simulink model "eVTOL_HIL"  (R2024b)
settings: Solver=FixedStepAuto  StartTime=0.0  StopTime=inf  FixedStep=SAMPLE_TIME  RelTol=1e-3
values from neighbouring files (symbols this model uses):
  aDl =     [initdata.mat]
  aDr =     [initdata.mat]
  aDyn =     [initdata.mat]
  aLat =     [initdata.mat]
  aLon =     [initdata.mat]
  D = Prop.D    [EOM_dt_MC.m]    (also in EOM_get_alf_dt_de_prop_evtol.m = CD * QS)
  General = init_layoutdata    [EOM_dt_MC.m]    (also in build_optimized_CA.m; initdata.mat = ; initdata_HIL_eVTOL.m)
  mass = Con(3)    [EOM_get_alf_dt_de_prop_evtol.m]    (also in initdata.mat = 2255.54; initdata_HIL_eVTOL.m = 7)
  Motor = init_motor_evtol    [EOM_dt_MC.m]    (also in initdata.mat = []; initdata_HIL_eVTOL.m)
  Prop = init_propeller_evtol_new    [EOM_dt_MC.m]    (also in initdata_HIL_eVTOL.m)
  SAMPLE_TIME = 0.01    [initdata_HIL_eVTOL.m]
undefined symbols (not defined in the file or in its folder): aDa, aDe, asbhl20env, Environment, InitData, magnitude
libraries: simulink_extras x16, vrlib x8, matrix_library x6, sharedutil x6, aerolibwindfilters x4, sharedtransform x4, aerolibfltsims x3, instrumentseriallib x3, uavmavlinklib x3, aerolibasang x3, aerolibobsolete x2, aerolibanimutils x1
(part 4 of 4)

== system eVTOL_HIL/eVTOL Dynamic Model/airframe/force moment/aero F&M in body axis/nonunit value ==
  V : Inport
  pqr : Inport  Port=2
  alphaDot : Inport  Port=3
  CA : Constant  Value=General.MAC
  Demux2 : Demux  Outputs=3
      settings: DisplayOption=none
  Gain : Gain  Gain=2  SaturateOnIntegerOverflow=on  OutDataTypeStr=Inherit: Same as input  ParamDataTypeStr=Inherit: Same as input
  Mux18 : Mux  Inputs=3
  Product{1..4} (4 alike) : Product  Inputs=/**  SaturateOnIntegerOverflow=on  OutDataTypeStr=Inherit: Same as first input
  b : Constant  Value=General.b
  pqr_n : Outport  VectorParamsAs1DForOutWhenUnconnected=off
  alphaDot_n : Outport  Port=2  VectorParamsAs1DForOutWhenUnconnected=off
  wires:
  pqr/1 -> Demux2/1
  V/1 -> Gain/1
  Product4/1 -> Mux18/2
  Product2/1 -> Mux18/3
  Gain/1 -> Product1/1, Product2/1, Product3/1, Product4/1
  b/1 -> Product1/2, Product2/2
  Demux2/3 -> Product2/3  "r"
  Demux2/2 -> Product4/3  "q"
  Demux2/1 -> Product1/3  "p"
  CA/1 -> Product4/2, Product3/2
  Mux18/1 -> pqr_n/1
  Product1/1 -> Mux18/1
  alphaDot/1 -> Product3/3
  Product3/1 -> alphaDot_n/1

== system eVTOL_HIL/eVTOL Dynamic Model/Environment/Wind Models/Dryden Wind Turbulence Model (Continuous (+q -r))/RMS turbulence intensities/High Altitude Intensity ==
  h : Inport
  Medium/High Altitude Intensity : Interpolation_n-D  Table=sigma_vec'  ExtrapMethod=Clip  ValidIndexMayReachLast=on  OutDataTypeStr=double
  PreLook-Up Index Search (altitude) : PreLookup  BreakpointsData=h_vec  BeginIndexSearchUsingPreviousIndexResult=on  UseLastBreakpoint=on  FractionDataTypeStr=double
  PreLook-Up Index Search (prob of exceed) : PreLookup  BreakpointsData=[1:7]  BeginIndexSearchUsingPreviousIndexResult=on  UseLastBreakpoint=on  FractionDataTypeStr=double
  Probability of Exceedance : Constant  Value=TurbProb
  sigma_ug sigma_vg sigma_wg : Outport  InitialOutput=0  VectorParamsAs1DForOutWhenUnconnected=off
  wires:
  PreLook-Up Index Search (prob of exceed)/2 -> Medium/High Altitude Intensity/4
  PreLook-Up Index Search (prob of exceed)/1 -> Medium/High Altitude Intensity/3
  PreLook-Up Index Search (altitude)/2 -> Medium/High Altitude Intensity/2
  PreLook-Up Index Search (altitude)/1 -> Medium/High Altitude Intensity/1
  h/1 -> PreLook-Up Index Search (altitude)/1
  Medium/High Altitude Intensity/1 -> sigma_ug sigma_vg sigma_wg/1
  Probability of Exceedance/1 -> PreLook-Up Index Search (prob of exceed)/1

== system eVTOL_HIL/eVTOL Dynamic Model/Environment/Wind Models/Dryden Wind Turbulence Model (Continuous (+q -r))/RMS turbulence intensities/Low Altitude Intensity ==
  Windspeed at 20ft (6m) : Inport
  h : Inport  Port=2
  Limit Height h<1000ft : Saturate  UpperLimit=max_height_low  LowerLimit=0
  Low Altitude Intensity : Fcn  Expr=1/(0.177+0.000823*u(1))^0.4
  "sigma_ug, sigma_vg" : Product  InputSameDT=on  SaturateOnIntegerOverflow=on  OutDataTypeStr=Inherit: Same as first input
  "sigma_wg " : Gain  Gain=0.1  SaturateOnIntegerOverflow=on  OutDataTypeStr=Inherit: Same as input  ParamDataTypeStr=Inherit: Same as input
  sigma_ug sigma_vg : Outport  InitialOutput=0  VectorParamsAs1DForOutWhenUnconnected=off
  sigma_wg : Outport  Port=2  InitialOutput=0  VectorParamsAs1DForOutWhenUnconnected=off
  wires:
  "sigma_ug, sigma_vg"/1 -> sigma_ug sigma_vg/1
  h/1 -> Limit Height h<1000ft/1
  Low Altitude Intensity/1 -> "sigma_ug, sigma_vg"/1
  "sigma_wg "/1 -> sigma_wg/1, "sigma_ug, sigma_vg"/2
  Windspeed at 20ft (6m)/1 -> "sigma_wg "/1
  Limit Height h<1000ft/1 -> Low Altitude Intensity/1

== system eVTOL_HIL/eVTOL Dynamic Model/Environment/Wind Models/Dryden Wind Turbulence Model (Continuous (+q -r))/Select angular rates/Interpolate rates ==
  pgw_h&l : Inport
  qgw_h&l : Inport  Port=2
  rgw_h&l : Inport  Port=3
  DCM : Inport  Port=4
  Wind direction : Inport  Port=5
  Altitude : Inport  Port=6
  Action Port : ActionPort  PropagateVarSize=During execution  ActionPortLabel=else
  Mux : Mux  Inputs=3
  Mux1 : Mux  Inputs=3
  Product1 : Product  Inputs=**/  SaturateOnIntegerOverflow=on  OutDataTypeStr=Inherit: Same as first input
  Selector : Selector  InputPortWidth=2  IndexOptions=Index vector (dialog)  Indices=1  OutputSizes=1
  Selector1 : Selector  InputPortWidth=2  IndexOptions=Index vector (dialog)  Indices=1  OutputSizes=1
  Selector2 : Selector  InputPortWidth=2  IndexOptions=Index vector (dialog)  Indices=1  OutputSizes=1
  Selector3 : Selector  InputPortWidth=2  IndexOptions=Index vector (dialog)  Indices=2  OutputSizes=1
  Selector4 : Selector  InputPortWidth=2  IndexOptions=Index vector (dialog)  Indices=2  OutputSizes=1
  Selector5 : Selector  InputPortWidth=2  IndexOptions=Index vector (dialog)  Indices=2  OutputSizes=1
  Sum : Sum  Inputs=|-+  SaturateOnIntegerOverflow=on
  Sum1 : Sum  Inputs=|+-  SaturateOnIntegerOverflow=on
  Sum2 : Sum  Inputs=-+|  SaturateOnIntegerOverflow=on
  Sum3 : Sum  Inputs=++|  SaturateOnIntegerOverflow=on
  max_height_low : Constant  Value=max_height_low
  min_height_high : Constant  Value=min_height_high
  wind to body transformation : Subsystem
  pgw,qgw,rgw : Outport  InitialOutput=0  VectorParamsAs1DForOutWhenUnconnected=off
  wires:
  Mux/1 -> wind to body transformation/3(pg_l,qg_l,rg_l)
  DCM/1 -> wind to body transformation/1(DCM)
  wind to body transformation/1(pg,qg,rg) -> Sum3/1, Sum2/1
  Sum3/1 -> pgw,qgw,rgw/1
  Product1/1 -> Sum3/2
  Mux1/1 -> Sum2/2
  Sum2/1 -> Product1/1
  Sum1/1 -> Product1/2
  Sum/1 -> Product1/3
  Altitude/1 -> Sum1/1
  min_height_high/1 -> Sum/2
  max_height_low/1 -> Sum1/2, Sum/1
  Wind direction/1 -> wind to body transformation/2(Wind direction)
  Selector3/1 -> Mux1/1
  Selector4/1 -> Mux1/2
  Selector5/1 -> Mux1/3
  pgw_h&l/1 -> Selector/1, Selector3/1
  qgw_h&l/1 -> Selector4/1, Selector1/1
  rgw_h&l/1 -> Selector5/1, Selector2/1
  Selector/1 -> Mux/1
  Selector1/1 -> Mux/2
  Selector2/1 -> Mux/3

== system eVTOL_HIL/eVTOL Dynamic Model/Environment/Wind Models/Dryden Wind Turbulence Model (Continuous (+q -r))/Select angular rates/Low altitude rates ==
  DCM : Inport
  pgw_h&l : Inport  Port=2
  qgw_h&l : Inport  Port=3
  rgw_h&l : Inport  Port=4
  Wind direction : Inport  Port=5
  Action Port : ActionPort  PropagateVarSize=During execution  ActionPortLabel=if(u1<=max_height_low)
  Mux : Mux  Inputs=3
  Selector : Selector  InputPortWidth=2  IndexOptions=Index vector (dialog)  Indices=1  OutputSizes=1
  Selector1 : Selector  InputPortWidth=2  IndexOptions=Index vector (dialog)  Indices=1  OutputSizes=1
  Selector2 : Selector  InputPortWidth=2  IndexOptions=Index vector (dialog)  Indices=1  OutputSizes=1
  wind to body transformation : Subsystem
  pgw,qgw,rgw : Outport  InitialOutput=0  VectorParamsAs1DForOutWhenUnconnected=off
  wires:
  DCM/1 -> wind to body transformation/1(DCM)
  pgw_h&l/1 -> Selector/1
  qgw_h&l/1 -> Selector1/1
  rgw_h&l/1 -> Selector2/1
  Selector/1 -> Mux/1
  Selector1/1 -> Mux/2
  Selector2/1 -> Mux/3
  Mux/1 -> wind to body transformation/3(pg_l,qg_l,rg_l)
  wind to body transformation/1(pg,qg,rg) -> pgw,qgw,rgw/1
  Wind direction/1 -> wind to body transformation/2(Wind direction)

== system eVTOL_HIL/eVTOL Dynamic Model/Environment/Wind Models/Dryden Wind Turbulence Model (Continuous (+q -r))/Select angular rates/Medium//High altitude rates ==
  pgw_h&l : Inport
  qgw_h&l : Inport  Port=2
  rgw_h&l : Inport  Port=3
  Action Port : ActionPort  PropagateVarSize=During execution  ActionPortLabel=elseif(u1>=min_height_high)
  Gain : Gain  SaturateOnIntegerOverflow=on  OutDataTypeStr=Inherit: Same as input  ParamDataTypeStr=Inherit: Same as input
  Mux : Mux  Inputs=3
  Selector3 : Selector  InputPortWidth=6  IndexOptions=Index vector (dialog)  Indices=[ 2 4 6]  OutputSizes=1
  pgw,qgw,rgw : Outport  InitialOutput=0  VectorParamsAs1DForOutWhenUnconnected=off
  wires:
  Gain/1 -> pgw,qgw,rgw/1
  Selector3/1 -> Gain/1
  pgw_h&l/1 -> Mux/1
  qgw_h&l/1 -> Mux/2
  rgw_h&l/1 -> Mux/3
  Mux/1 -> Selector3/1

== system eVTOL_HIL/eVTOL Dynamic Model/Environment/Wind Models/Dryden Wind Turbulence Model (Continuous (+q -r))/Select angular rates/Merge Subsystems ==
  low : Inport
  high : Inport  Port=2
  interpolated : Inport  Port=3
  Demux : Demux  Outputs=3
      settings: DisplayOption=none
  Merge : Merge  Inputs=3
  pgw : Outport  VectorParamsAs1DForOutWhenUnconnected=off
  qgw : Outport  Port=2  VectorParamsAs1DForOutWhenUnconnected=off
  rgw : Outport  Port=3  VectorParamsAs1DForOutWhenUnconnected=off
  wires:
  low/1 -> Merge/1
  high/1 -> Merge/2
  interpolated/1 -> Merge/3
  Demux/2 -> qgw/1
  Demux/3 -> rgw/1
  Demux/1 -> pgw/1
  Merge/1 -> Demux/1

== system eVTOL_HIL/eVTOL Dynamic Model/Environment/Wind Models/Dryden Wind Turbulence Model (Continuous (+q -r))/Select velocities/Interpolate velocities ==
  ugw_h&l : Inport
  vgw_h&l : Inport  Port=2
  wgw_h&l : Inport  Port=3
  DCM : Inport  Port=4
  Wind direction : Inport  Port=5
  Altitude : Inport  Port=6
  Action Port : ActionPort  PropagateVarSize=During execution  ActionPortLabel=else
  Mux : Mux  Inputs=3
  Mux1 : Mux  Inputs=3
  Product1 : Product  Inputs=**/  SaturateOnIntegerOverflow=on  OutDataTypeStr=Inherit: Same as first input
  Selector : Selector  InputPortWidth=2  IndexOptions=Index vector (dialog)  Indices=1  OutputSizes=1
  Selector1 : Selector  InputPortWidth=2  IndexOptions=Index vector (dialog)  Indices=1  OutputSizes=1
  Selector2 : Selector  InputPortWidth=2  IndexOptions=Index vector (dialog)  Indices=1  OutputSizes=1
  Selector3 : Selector  InputPortWidth=2  IndexOptions=Index vector (dialog)  Indices=2  OutputSizes=1
  Selector4 : Selector  InputPortWidth=2  IndexOptions=Index vector (dialog)  Indices=2  OutputSizes=1
  Selector5 : Selector  InputPortWidth=2  IndexOptions=Index vector (dialog)  Indices=2  OutputSizes=1
  Sum : Sum  Inputs=|-+  SaturateOnIntegerOverflow=on
  Sum1 : Sum  Inputs=|+-  SaturateOnIntegerOverflow=on
  Sum2 : Sum  Inputs=-+|  SaturateOnIntegerOverflow=on
  Sum3 : Sum  Inputs=++|  SaturateOnIntegerOverflow=on
  max_height_low : Constant  Value=max_height_low
  min_height_high : Constant  Value=min_height_high
  wind to body transformation : Subsystem
  ugw,vgw,wgw : Outport  InitialOutput=0  VectorParamsAs1DForOutWhenUnconnected=off
  wires:
  Mux/1 -> wind to body transformation/3(ug_l,vg_l,wg_l)
  Wind direction/1 -> wind to body transformation/2(Wind direction)
  DCM/1 -> wind to body transformation/1(DCM)
  wind to body transformation/1(ug,vg,wg) -> Sum3/1, Sum2/1
  Sum3/1 -> ugw,vgw,wgw/1
  Product1/1 -> Sum3/2
  Mux1/1 -> Sum2/2
  Sum2/1 -> Product1/1
  Sum1/1 -> Product1/2
  Sum/1 -> Product1/3
  Altitude/1 -> Sum1/1
  min_height_high/1 -> Sum/2
  max_height_low/1 -> Sum1/2, Sum/1
  Selector3/1 -> Mux1/1
  Selector4/1 -> Mux1/2
  Selector5/1 -> Mux1/3
  ugw_h&l/1 -> Selector/1, Selector3/1
  vgw_h&l/1 -> Selector4/1, Selector1/1
  wgw_h&l/1 -> Selector5/1, Selector2/1
  Selector/1 -> Mux/1
  Selector1/1 -> Mux/2
  Selector2/1 -> Mux/3

== system eVTOL_HIL/eVTOL Dynamic Model/Environment/Wind Models/Dryden Wind Turbulence Model (Continuous (+q -r))/Select velocities/Low altitude velocities ==
  DCM : Inport
  ugw_h&l : Inport  Port=2
  vgw_h&l : Inport  Port=3
  wgw_h&l : Inport  Port=4
  Wind direction : Inport  Port=5
  Action Port : ActionPort  PropagateVarSize=During execution  ActionPortLabel=if(u1<=max_height_low)
  Mux : Mux  Inputs=3
  Selector : Selector  InputPortWidth=2  IndexOptions=Index vector (dialog)  Indices=1  OutputSizes=1
  Selector1 : Selector  InputPortWidth=2  IndexOptions=Index vector (dialog)  Indices=1  OutputSizes=1
  Selector2 : Selector  InputPortWidth=2  IndexOptions=Index vector (dialog)  Indices=1  OutputSizes=1
  wind to body transformation : Subsystem
  ugw,vgw,wgw : Outport  InitialOutput=0  VectorParamsAs1DForOutWhenUnconnected=off
  wires:
  Mux/1 -> wind to body transformation/3(ug_l,vg_l,wg_l)
  Selector2/1 -> Mux/3
  wind to body transformation/1(ug,vg,wg) -> ugw,vgw,wgw/1
  Wind direction/1 -> wind to body transformation/2(Wind direction)
  DCM/1 -> wind to body transformation/1(DCM)
  Selector1/1 -> Mux/2
  Selector/1 -> Mux/1
  wgw_h&l/1 -> Selector2/1
  vgw_h&l/1 -> Selector1/1
  ugw_h&l/1 -> Selector/1

== system eVTOL_HIL/eVTOL Dynamic Model/Environment/Wind Models/Dryden Wind Turbulence Model (Continuous (+q -r))/Select velocities/Medium//High altitude velocities ==
  ugw_h&l : Inport
  vgw_h&l : Inport  Port=2
  wgw_h&l : Inport  Port=3
  Action Port : ActionPort  PropagateVarSize=During execution  ActionPortLabel=elseif(u1>=min_height_high)
  Gain : Gain  SaturateOnIntegerOverflow=on  OutDataTypeStr=Inherit: Same as input  ParamDataTypeStr=Inherit: Same as input
  Mux : Mux  Inputs=3
  Selector3 : Selector  InputPortWidth=6  IndexOptions=Index vector (dialog)  Indices=[ 2 4 6]  OutputSizes=1
  ugw,vgw,wgw : Outport  InitialOutput=0  VectorParamsAs1DForOutWhenUnconnected=off
  wires:
  vgw_h&l/1 -> Mux/2
  Gain/1 -> ugw,vgw,wgw/1
  Selector3/1 -> Gain/1
  Mux/1 -> Selector3/1
  wgw_h&l/1 -> Mux/3
  ugw_h&l/1 -> Mux/1

== system eVTOL_HIL/eVTOL Dynamic Model/Environment/Wind Models/Dryden Wind Turbulence Model (Continuous (+q -r))/Select velocities/Merge Subsystems ==
  low : Inport
  high : Inport  Port=2
  interpolated : Inport  Port=3
  Demux : Demux  Outputs=3
      settings: DisplayOption=none
  Merge : Merge  Inputs=3
  ugw : Outport  VectorParamsAs1DForOutWhenUnconnected=off
  vgw : Outport  Port=2  VectorParamsAs1DForOutWhenUnconnected=off
  wgw : Outport  Port=3  VectorParamsAs1DForOutWhenUnconnected=off
  wires:
  Merge/1 -> Demux/1
  Demux/1 -> ugw/1
  Demux/3 -> wgw/1
  Demux/2 -> vgw/1
  interpolated/1 -> Merge/3
  high/1 -> Merge/2
  low/1 -> Merge/1

== system eVTOL_HIL/eVTOL Dynamic Model/Environment/Wind Models/Dryden Wind Turbulence Model (Continuous (+q -r))/Turbulence scale lengths/Low altitude scale length ==
  h : Inport
  Limit Function 10ft to 1000ft : Saturate  UpperLimit=max_height_low  LowerLimit=10
  Low Altitude Scale Length : Fcn  Expr=u(1)/(0.177+0.000823*u(1))^1.2
  L_ug L_vg : Outport  InitialOutput=0  VectorParamsAs1DForOutWhenUnconnected=off
  L_wg : Outport  Port=2  InitialOutput=0  VectorParamsAs1DForOutWhenUnconnected=off
  wires:
  h/1 -> Limit Function 10ft to 1000ft/1
  Low Altitude Scale Length/1 -> L_ug L_vg/1
  Limit Function 10ft to 1000ft/1 -> L_wg/1, Low Altitude Scale Length/1

== system eVTOL_HIL/eVTOL Dynamic Model/Environment/Wind Models/Dryden Wind Turbulence Model (Continuous (+q -r))/Turbulence scale lengths/Medium//High altitude scale length ==
  Length Conversion : Subsystem
  Medium/High Altitude : Constant  Value=L_high
  L_ug L_vg L_wg : Outport  Unit=ft  InitialOutput=0  VectorParamsAs1DForOutWhenUnconnected=off
  wires:
  Medium/High Altitude/1 -> Length Conversion/1(in)
  Length Conversion/1(out) -> L_ug L_vg L_wg/1

== system eVTOL_HIL/eVTOL Dynamic Model/airframe/force moment/aero F&M in body axis/Aerodynamic Coefficients/Actuator Increments ==
  Actuators : Inport
  incid : Inport  Port=2
  Aileron : Subsystem
  Bus Selector1 : BusSelector  OutputSignals=dl,dr,da
  Demux : Demux  Outputs=2
  Reshape : Reshape
  Sum : Sum  Inputs=+++
  Terminator : Terminator
  V_left : Subsystem
  V_right : Subsystem
  cl : Outport  InitialOutput=0  VectorParamsAs1DForOutWhenUnconnected=off
  wires:
  Actuators/1 -> Bus Selector1/1
  Sum/1 -> Reshape/1
  V_right/1(dr_Coeff) -> Sum/2
  V_left/1(dl_Coeff) -> Sum/1
  Bus Selector1/1 -> V_left/2(dl)  "<dl>"
  Bus Selector1/3 -> Aileron/2(da)  "<da>"
  incid/1 -> Demux/1
  Demux/1 -> Aileron/1(alpha), V_right/1(alpha), V_left/1(alpha)  "alpha"
  Demux/2 -> Terminator/1  "beta"
  Aileron/1(da_Coeff) -> Sum/3
  Bus Selector1/2 -> V_right/2(dr)  "<dr>"
  Reshape/1 -> cl/1

== system eVTOL_HIL/eVTOL Dynamic Model/airframe/force moment/aero F&M in body axis/Aerodynamic Coefficients/Basic Coefficients ==
  Incid : Inport
  mach : Inport  Port=2
  2-D Lookup Table : Lookup_n-D  NumberOfTableDimensions=1  BreakpointsForDimension1=aLon.alpha  BreakpointsForDimension2=aLon.mach  BreakpointsForDimension3=aLon.flap  Table=aLon.CL  InternalRulePriority=Speed  RndMeth=Simplest
  2-D Lookup Table1 : Lookup_n-D  NumberOfTableDimensions=1  BreakpointsForDimension1=aLon.alpha  BreakpointsForDimension2=aLon.mach  BreakpointsForDimension3=aLon.flap  Table=aLon.CD  InternalRulePriority=Speed  RndMeth=Simplest
  2-D Lookup Table2 : Lookup_n-D  NumberOfTableDimensions=1  BreakpointsForDimension1=aLon.alpha  BreakpointsForDimension2=aLon.mach  BreakpointsForDimension3=aLon.flap  Table=aLon.Cm  InternalRulePriority=Speed  RndMeth=Simplest
  2-D Lookup Table3 : Lookup_n-D  BreakpointsForDimension1=aLat.beta  BreakpointsForDimension2=aLat.alpha  BreakpointsForDimension3=aLat.mach  Table=aLat.dCD  InternalRulePriority=Speed  RndMeth=Simplest
      settings: InputPortMap=u0,u1
  2-D Lookup Table4 : Lookup_n-D  BreakpointsForDimension1=aLat.beta  BreakpointsForDimension2=aLat.alpha  BreakpointsForDimension3=aLat.mach  Table=aLat.dCY  InternalRulePriority=Speed  RndMeth=Simplest
      settings: InputPortMap=u0,u1
  2-D Lookup Table5 : Lookup_n-D  BreakpointsForDimension1=aLat.beta  BreakpointsForDimension2=aLat.alpha  BreakpointsForDimension3=aLat.mach  Table=aLat.dCl  InternalRulePriority=Speed  RndMeth=Simplest
      settings: InputPortMap=u0,u1
  2-D Lookup Table6 : Lookup_n-D  BreakpointsForDimension1=aLat.beta  BreakpointsForDimension2=aLat.alpha  BreakpointsForDimension3=aLat.mach  Table=aLat.dCL  InternalRulePriority=Speed  RndMeth=Simplest
      settings: InputPortMap=u0,u1
  2-D Lookup Table7 : Lookup_n-D  BreakpointsForDimension1=aLat.beta  BreakpointsForDimension2=aLat.alpha  BreakpointsForDimension3=aLat.mach  Table=aLat.dCm  InternalRulePriority=Speed  RndMeth=Simplest
      settings: InputPortMap=u0,u1
  2-D Lookup Table8 : Lookup_n-D  BreakpointsForDimension1=aLat.beta  BreakpointsForDimension2=aLat.alpha  BreakpointsForDimension3=aLat.mach  Table=aLat.dCn  InternalRulePriority=Speed  RndMeth=Simplest
      settings: InputPortMap=u0,u1
  Constant1 : Constant  Value=0
  Demux : Demux  Outputs=2
  Display : Display
  Display1 : Display
  Gain : Gain
  Mux1 : Mux  Inputs=6
  Mux2 : Mux  Inputs=6
  Reshape : Reshape
  Saturation : Saturate  UpperLimit=0.1  LowerLimit=0
  Scope{1..5} (5 alike) : Scope
  Sum5 : Sum  Inputs=+++  InputSameDT=on  SaturateOnIntegerOverflow=on  OutDataTypeStr=Inherit: Same as first input
  cl : Outport  InitialOutput=0  VectorParamsAs1DForOutWhenUnconnected=off
  wires:
  Mux1/1 -> Display/1, Sum5/2
  Demux/1 -> Scope5/1, [alpha]  "alpha"
  Demux/2 -> [beta]  "beta"
  2-D Lookup Table1/1 -> Mux1/2, Scope3/1  "CD"
  Constant1/1 -> Mux1/6, Mux1/4, Mux1/3
  2-D Lookup Table4/1 -> Mux2/3  "dCY"
  2-D Lookup Table5/1 -> Mux2/4  "dCl"
  2-D Lookup Table8/1 -> Mux2/6  "dCn"
  Sum5/1 -> Reshape/1
  Mux2/1 -> Sum5/3, Display1/1
  Incid/1 -> Demux/1
  [alpha] -> 2-D Lookup Table/1, Scope4/1
  2-D Lookup Table/1 -> Scope2/1, Mux1/1  "CL"
  [alpha] -> 2-D Lookup Table1/1
  [alpha] -> 2-D Lookup Table2/1
  2-D Lookup Table2/1 -> Gain/1  "Cm"
  [beta] -> 2-D Lookup Table6/1
  2-D Lookup Table6/1 -> Mux2/1  "dCL"
  [alpha] -> 2-D Lookup Table6/2
  [alpha] -> 2-D Lookup Table3/2
  [beta] -> 2-D Lookup Table3/1
  2-D Lookup Table3/1 -> Mux2/2  "dCD"
  [beta] -> 2-D Lookup Table4/1
  [alpha] -> 2-D Lookup Table4/2
  [alpha] -> 2-D Lookup Table5/2
  [beta] -> 2-D Lookup Table5/1
  [beta] -> 2-D Lookup Table7/1
  [alpha] -> 2-D Lookup Table7/2
  2-D Lookup Table7/1 -> Mux2/5  "dCm"
  [alpha] -> 2-D Lookup Table8/2
  [beta] -> 2-D Lookup Table8/1
  Saturation/1 -> Scope1/1, [mach]
  mach/1 -> Saturation/1
  Gain/1 -> Mux1/5
  Reshape/1 -> cl/1

== system eVTOL_HIL/eVTOL Dynamic Model/airframe/force moment/aero F&M in body axis/Aerodynamic Coefficients/Body Rate Damping ==
  Incid : Inport
  pqrn : Inport  Port=2
  alphaDot_n : Inport  Port=3
  1-D Lookup Table : Lookup_n-D  NumberOfTableDimensions=1  BreakpointsForDimension1=aDyn.alpha  BreakpointsForDimension2=aDyn.flap  Table=aDyn.CYp  InternalRulePriority=Speed  RndMeth=Simplest
  1-D Lookup Table1 : Lookup_n-D  NumberOfTableDimensions=1  BreakpointsForDimension1=aDyn.alpha  BreakpointsForDimension2=aDyn.flap  Table=aDyn.Clp  InternalRulePriority=Speed  RndMeth=Simplest
  1-D Lookup Table2 : Lookup_n-D  NumberOfTableDimensions=1  BreakpointsForDimension1=aDyn.alpha  BreakpointsForDimension2=aDyn.flap  Table=aDyn.Cnp  InternalRulePriority=Speed  RndMeth=Simplest
  1-D Lookup Table3 : Lookup_n-D  NumberOfTableDimensions=1  BreakpointsForDimension1=aDyn.alpha  BreakpointsForDimension2=aDyn.flap  Table=aDyn.CYr  InternalRulePriority=Speed  RndMeth=Simplest
  1-D Lookup Table4 : Lookup_n-D  NumberOfTableDimensions=1  BreakpointsForDimension1=aDyn.alpha  BreakpointsForDimension2=aDyn.flap  Table=aDyn.Clr  InternalRulePriority=Speed  RndMeth=Simplest
  1-D Lookup Table5 : Lookup_n-D  NumberOfTableDimensions=1  BreakpointsForDimension1=aDyn.alpha  BreakpointsForDimension2=aDyn.flap  Table=aDyn.Cnr  InternalRulePriority=Speed  RndMeth=Simplest
  1-D Lookup Table6 : Lookup_n-D  NumberOfTableDimensions=1  BreakpointsForDimension1=aDyn.alpha  BreakpointsForDimension2=aDyn.flap  Table=aDyn.CLq  InternalRulePriority=Speed  RndMeth=Simplest
  1-D Lookup Table7 : Lookup_n-D  NumberOfTableDimensions=1  BreakpointsForDimension1=aDyn.alpha  BreakpointsForDimension2=aDyn.flap  Table=aDyn.Cmq  InternalRulePriority=Speed  RndMeth=Simplest
  1-D Lookup Table8 : Lookup_n-D  NumberOfTableDimensions=1  BreakpointsForDimension1=aDyn.alpha  BreakpointsForDimension2=aDyn.flap  Table=aDyn.CLAlphaDot  InternalRulePriority=Speed  RndMeth=Simplest
  1-D Lookup Table9 : Lookup_n-D  NumberOfTableDimensions=1  BreakpointsForDimension1=aDyn.alpha  BreakpointsForDimension2=aDyn.flap  Table=aDyn.CmAlphaDot  InternalRulePriority=Speed  RndMeth=Simplest
  Add : Sum  Inputs=++++
  Constant{,6..7,13} (4 alike) : Constant  Value=0
  Demux : Demux  Outputs=3
  Demux1 : Demux  Outputs=2
  Mux{1..4} (4 alike) : Mux  Inputs=6
  Product{4..7} (4 alike) : Product  InputSameDT=on  SaturateOnIntegerOverflow=on  OutDataTypeStr=Inherit: Same as first input
  Reshape : Reshape
  Terminator : Terminator
  cl : Outport  InitialOutput=0  VectorParamsAs1DForOutWhenUnconnected=off
  wires:
  Add/1 -> Reshape/1
  1-D Lookup Table/1 -> Mux1/3  "CYp"
  1-D Lookup Table2/1 -> Mux1/6  "Cnp"
  Mux1/1 -> Product4/1
  1-D Lookup Table1/1 -> Mux1/4  "Clp"
  pqrn/1 -> Demux/1
  Demux/1 -> [p]
  Demux/2 -> [q]
  Demux/3 -> [r]
  Constant/1 -> Mux1/1, Mux1/2, Mux1/5
  1-D Lookup Table7/1 -> Mux2/5  "Cmq"
  1-D Lookup Table6/1 -> Mux2/1  "CLq"
  Mux2/1 -> Product5/1
  1-D Lookup Table3/1 -> Mux3/3  "CYr"
  Mux3/1 -> Product6/1
  1-D Lookup Table4/1 -> Mux3/4  "Clr"
  1-D Lookup Table5/1 -> Mux3/6  "Cnr"
  Constant7/1 -> Mux3/2, Mux3/5, Mux3/1
  Constant13/1 -> Mux4/6, Mux4/4, Mux4/3, Mux4/2
  1-D Lookup Table9/1 -> Mux4/5  "CmAlphaDot"
  1-D Lookup Table8/1 -> Mux4/1  "CLAlphaDot"
  Constant6/1 -> Mux2/4, Mux2/6, Mux2/3, Mux2/2
  Mux4/1 -> Product7/1
  Product4/1 -> Add/1
  Product7/1 -> Add/4
  Demux1/2 -> Terminator/1  "beta"
  Demux1/1 -> [alpha]  "alpha"
  Incid/1 -> Demux1/1
  Product5/1 -> Add/3
  [alpha] -> 1-D Lookup Table3/1, 1-D Lookup Table4/1, 1-D Lookup Table9/1, 1-D Lookup Table8/1, 1-D Lookup Table7/1, 1-D Lookup Table6/1, 1-D Lookup Table5/1, 1-D Lookup Table2/1, 1-D Lookup Table1/1, 1-D Lookup Table/1
  Product6/1 -> Add/2
  Reshape/1 -> cl/1
  [r] -> Product6/2
  [q] -> Product5/2
  alphaDot_n/1 -> Product7/2
  [p] -> Product4/2

== system eVTOL_HIL/eVTOL Dynamic Model/airframe/force moment/aero F&M in body axis/Aerodynamic Coefficients/CLCDCY-CXCYCZ ==
  Incid : Inport
  Cl_LDY : Inport  Port=2
  Cl_xA : Fcn  Expr=-u[4]*cos(u[2])*cos(u[1])+u[3]*sin(u[1])
  Cl_yA : Fcn  Expr=-u[4]*sin(u[2])+u[5]
  Cl_zA : Fcn  Expr=-u[4]*cos(u[2])*sin(u[1])-u[3]*cos(u[1])
  Mux : Mux  Inputs=3
  Mux1 : Mux  Inputs=2
  Cl_XYZ : Outport  VectorParamsAs1DForOutWhenUnconnected=off
  wires:
  Mux/1 -> Cl_XYZ/1
  Cl_LDY/1 -> Mux1/2
  Incid/1 -> Mux1/1
  Cl_zA/1 -> Mux/3
  Cl_yA/1 -> Mux/2
  Cl_xA/1 -> Mux/1
  Mux1/1 -> Cl_zA/1, Cl_yA/1, Cl_xA/1

== system eVTOL_HIL/eVTOL Dynamic Model/Environment/Wind Models/Dryden Wind Turbulence Model (Continuous (+q -r))/Select angular rates/Interpolate rates/wind to body transformation ==
  DCM : Inport
  Wind direction : Inport  Port=2
  pg_l,qg_l,rg_l : Inport  Port=3
  Demux : Demux  Outputs=3
      settings: DisplayOption=none
  Product : Product  Multiplication=Matrix(*)  SaturateOnIntegerOverflow=on  OutDataTypeStr=Inherit: Same as first input
  Reshape : Reshape  OutputDimensionality=Customize  OutputDimensions=[3,1]
  Reshape1 : Reshape
  Vector Concatenate : Concatenate  NumInputs=3
  convert to earth coords : Subsystem
  pg,qg,rg : Outport  VectorParamsAs1DForOutWhenUnconnected=off
  wires:
  Reshape1/1 -> pg,qg,rg/1
  Reshape/1 -> Product/2
  DCM/1 -> Product/1
  Wind direction/1 -> convert to earth coords/1(Wind direction)
  convert to earth coords/1(pg) -> Vector Concatenate/1
  convert to earth coords/2(qg) -> Vector Concatenate/2
  Vector Concatenate/1 -> Reshape/1
  Demux/1 -> convert to earth coords/2(pg_l)
  Demux/2 -> convert to earth coords/3(qg_l)
  Demux/3 -> Vector Concatenate/3
  Product/1 -> Reshape1/1
  pg_l,qg_l,rg_l/1 -> Demux/1

== system eVTOL_HIL/eVTOL Dynamic Model/Environment/Wind Models/Dryden Wind Turbulence Model (Continuous (+q -r))/Select angular rates/Low altitude rates/wind to body transformation ==
  DCM : Inport
  Wind direction : Inport  Port=2
  pg_l,qg_l,rg_l : Inport  Port=3
  Demux : Demux  Outputs=3
      settings: DisplayOption=none
  Product : Product  Multiplication=Matrix(*)  SaturateOnIntegerOverflow=on  OutDataTypeStr=Inherit: Same as first input
  Reshape : Reshape  OutputDimensionality=Column vector (2-D)
  Reshape1 : Reshape
  Vector Concatenate : Concatenate  NumInputs=3
  convert to earth coords : Subsystem
  pg,qg,rg : Outport  VectorParamsAs1DForOutWhenUnconnected=off
  wires:
  pg_l,qg_l,rg_l/1 -> Demux/1
  Product/1 -> Reshape1/1
  Demux/3 -> Vector Concatenate/3
  Demux/2 -> convert to earth coords/3(qg_l)
  Demux/1 -> convert to earth coords/2(pg_l)
  Vector Concatenate/1 -> Reshape/1
  convert to earth coords/2(qg) -> Vector Concatenate/2
  convert to earth coords/1(pg) -> Vector Concatenate/1
  Wind direction/1 -> convert to earth coords/1(Wind direction)
  DCM/1 -> Product/1
  Reshape/1 -> Product/2
  Reshape1/1 -> pg,qg,rg/1

== system eVTOL_HIL/eVTOL Dynamic Model/Environment/Wind Models/Dryden Wind Turbulence Model (Continuous (+q -r))/Select velocities/Interpolate velocities/wind to body transformation ==
  DCM : Inport
  Wind direction : Inport  Port=2
  ug_l,vg_l,wg_l : Inport  Port=3
  Demux : Demux  Outputs=3
      settings: DisplayOption=none
  Product : Product  Multiplication=Matrix(*)  SaturateOnIntegerOverflow=on  OutDataTypeStr=Inherit: Same as first input
  Reshape : Reshape  OutputDimensionality=Customize  OutputDimensions=[3,1]
  Reshape1 : Reshape
  Vector Concatenate : Concatenate  NumInputs=3
  convert to earth coords : Subsystem
  ug,vg,wg : Outport  VectorParamsAs1DForOutWhenUnconnected=off
  wires:
  Reshape1/1 -> ug,vg,wg/1
  Reshape/1 -> Product/2
  ug_l,vg_l,wg_l/1 -> Demux/1
  Product/1 -> Reshape1/1
  Demux/3 -> Vector Concatenate/3
  Demux/2 -> convert to earth coords/3(vg_l)
  Demux/1 -> convert to earth coords/2(ug_l)
  Vector Concatenate/1 -> Reshape/1
  convert to earth coords/2(vg) -> Vector Concatenate/2
  convert to earth coords/1(ug) -> Vector Concatenate/1
  Wind direction/1 -> convert to earth coords/1(Wind direction)
  DCM/1 -> Product/1

== system eVTOL_HIL/eVTOL Dynamic Model/Environment/Wind Models/Dryden Wind Turbulence Model (Continuous (+q -r))/Select velocities/Low altitude velocities/wind to body transformation ==
  DCM : Inport
  Wind direction : Inport  Port=2
  ug_l,vg_l,wg_l : Inport  Port=3
  Demux : Demux  Outputs=3
      settings: DisplayOption=none
  Product : Product  Multiplication=Matrix(*)  SaturateOnIntegerOverflow=on  OutDataTypeStr=Inherit: Same as first input
  Reshape : Reshape  OutputDimensionality=Column vector (2-D)
  Reshape1 : Reshape
  Vector Concatenate : Concatenate  NumInputs=3
  convert to earth coords : Subsystem
  ug,vg,wg : Outport  VectorParamsAs1DForOutWhenUnconnected=off
  wires:
  DCM/1 -> Product/1
  Wind direction/1 -> convert to earth coords/1(Wind direction)
  convert to earth coords/1(ug) -> Vector Concatenate/1
  convert to earth coords/2(vg) -> Vector Concatenate/2
  Vector Concatenate/1 -> Reshape/1
  Demux/1 -> convert to earth coords/2(ug_l)
  Demux/2 -> convert to earth coords/3(vg_l)
  Demux/3 -> Vector Concatenate/3
  Product/1 -> Reshape1/1
  ug_l,vg_l,wg_l/1 -> Demux/1
  Reshape/1 -> Product/2
  Reshape1/1 -> ug,vg,wg/1

== system eVTOL_HIL/eVTOL Dynamic Model/Environment/Wind Models/Dryden Wind Turbulence Model (Continuous (+q -r))/Turbulence scale lengths/Medium//High altitude scale length/Length Conversion ==
  in : Inport  Unit=m
  Unit Conversion : UnitConversion
  out : Outport  VectorParamsAs1DForOutWhenUnconnected=off
  wires:
  in/1 -> Unit Conversion/1
  Unit Conversion/1 -> out/1

== system eVTOL_HIL/eVTOL Dynamic Model/airframe/force moment/aero F&M in body axis/Aerodynamic Coefficients/Actuator Increments/Aileron ==
  alpha : Inport
  da : Inport  Port=2
  2-D Lookup Table3 : Lookup_n-D  NumberOfTableDimensions=1  BreakpointsForDimension1=aDa.alpha  BreakpointsForDimension2=aDe.alpha  BreakpointsForDimension3=aDe.flap  Table=aDa.CYDa  InternalRulePriority=Speed  RndMeth=Simplest
  2-D Lookup Table4 : Lookup_n-D  NumberOfTableDimensions=1  BreakpointsForDimension1=aDa.alpha  BreakpointsForDimension2=aDe.alpha  BreakpointsForDimension3=aDe.flap  Table=aDa.ClDa  InternalRulePriority=Speed  RndMeth=Simplest
  2-D Lookup Table5 : Lookup_n-D  NumberOfTableDimensions=1  BreakpointsForDimension1=aDa.alpha  BreakpointsForDimension2=aDe.alpha  BreakpointsForDimension3=aDe.flap  Table=aDa.CnDa  InternalRulePriority=Speed  RndMeth=Simplest
  Constant : Constant  Value=0
  Divide2 : Product  Inputs=**
  Divide3 : Product  Inputs=**
  Divide5 : Product  Inputs=**
  Mux1 : Mux  Inputs=6
  da_Coeff : Outport  VectorParamsAs1DForOutWhenUnconnected=off
  wires:
  alpha/1 -> 2-D Lookup Table5/1, 2-D Lookup Table4/1, 2-D Lookup Table3/1
  Mux1/1 -> da_Coeff/1
  da/1 -> Divide5/1, Divide3/1, Divide2/1
  Divide2/1 -> Mux1/3
  Divide3/1 -> Mux1/4
  2-D Lookup Table3/1 -> Divide2/2
  Divide5/1 -> Mux1/6
  2-D Lookup Table5/1 -> Divide5/2
  2-D Lookup Table4/1 -> Divide3/2
  Constant/1 -> Mux1/5, Mux1/2, Mux1/1

== system eVTOL_HIL/eVTOL Dynamic Model/airframe/force moment/aero F&M in body axis/Aerodynamic Coefficients/Actuator Increments/V_left ==
  alpha : Inport
  dl : Inport  Port=2
  2-D Lookup Table : Lookup_n-D  NumberOfTableDimensions=1  BreakpointsForDimension1=aDl.alpha  BreakpointsForDimension2=aDl.alpha  BreakpointsForDimension3=aDe.flap  Table=aDl.CLDl  InternalRulePriority=Speed  RndMeth=Simplest
  2-D Lookup Table1 : Lookup_n-D  NumberOfTableDimensions=1  BreakpointsForDimension1=aDl.alpha  BreakpointsForDimension2=aDe.alpha  BreakpointsForDimension3=aDe.flap  Table=aDl.CmDl  InternalRulePriority=Speed  RndMeth=Simplest
  2-D Lookup Table2 : Lookup_n-D  NumberOfTableDimensions=1  BreakpointsForDimension1=aDl.alpha  BreakpointsForDimension2=aDe.alpha  BreakpointsForDimension3=aDe.flap  Table=aDl.CDDl  InternalRulePriority=Speed  RndMeth=Simplest
  2-D Lookup Table3 : Lookup_n-D  NumberOfTableDimensions=1  BreakpointsForDimension1=aDl.alpha  BreakpointsForDimension2=aDe.alpha  BreakpointsForDimension3=aDe.flap  Table=aDl.CYDl  InternalRulePriority=Speed  RndMeth=Simplest
  2-D Lookup Table4 : Lookup_n-D  NumberOfTableDimensions=1  BreakpointsForDimension1=aDl.alpha  BreakpointsForDimension2=aDe.alpha  BreakpointsForDimension3=aDe.flap  Table=aDl.ClDl  InternalRulePriority=Speed  RndMeth=Simplest
  2-D Lookup Table5 : Lookup_n-D  NumberOfTableDimensions=1  BreakpointsForDimension1=aDl.alpha  BreakpointsForDimension2=aDe.alpha  BreakpointsForDimension3=aDe.flap  Table=aDl.CnDl  InternalRulePriority=Speed  RndMeth=Simplest
  Divide{,1..5} (6 alike) : Product  Inputs=**
  Mux1 : Mux  Inputs=6
  dl_Coeff : Outport  VectorParamsAs1DForOutWhenUnconnected=off
  wires:
  2-D Lookup Table/1 -> Divide/2
  2-D Lookup Table2/1 -> Divide1/2
  2-D Lookup Table1/1 -> Divide4/2
  Mux1/1 -> dl_Coeff/1
  Divide4/1 -> Mux1/5
  Divide/1 -> Mux1/1
  Divide1/1 -> Mux1/2
  Divide2/1 -> Mux1/3
  2-D Lookup Table3/1 -> Divide2/2
  Divide3/1 -> Mux1/4
  2-D Lookup Table4/1 -> Divide3/2
  dl/1 -> Divide5/1, Divide4/1, Divide3/1, Divide2/1, Divide1/1, Divide/1
  alpha/1 -> 2-D Lookup Table5/1, 2-D Lookup Table1/1, 2-D Lookup Table4/1, 2-D Lookup Table3/1, 2-D Lookup Table2/1, 2-D Lookup Table/1
  2-D Lookup Table5/1 -> Divide5/2
  Divide5/1 -> Mux1/6

== system eVTOL_HIL/eVTOL Dynamic Model/airframe/force moment/aero F&M in body axis/Aerodynamic Coefficients/Actuator Increments/V_right ==
  alpha : Inport
  dr : Inport  Port=2
  2-D Lookup Table : Lookup_n-D  NumberOfTableDimensions=1  BreakpointsForDimension1=aDr.alpha  BreakpointsForDimension2=aDl.alpha  BreakpointsForDimension3=aDe.flap  Table=aDr.CLDr  InternalRulePriority=Speed  RndMeth=Simplest
  2-D Lookup Table1 : Lookup_n-D  NumberOfTableDimensions=1  BreakpointsForDimension1=aDr.alpha  BreakpointsForDimension2=aDe.alpha  BreakpointsForDimension3=aDe.flap  Table=aDr.CmDr  InternalRulePriority=Speed  RndMeth=Simplest
  2-D Lookup Table2 : Lookup_n-D  NumberOfTableDimensions=1  BreakpointsForDimension1=aDr.alpha  BreakpointsForDimension2=aDe.alpha  BreakpointsForDimension3=aDe.flap  Table=aDr.CDDr  InternalRulePriority=Speed  RndMeth=Simplest
  2-D Lookup Table3 : Lookup_n-D  NumberOfTableDimensions=1  BreakpointsForDimension1=aDr.alpha  BreakpointsForDimension2=aDe.alpha  BreakpointsForDimension3=aDe.flap  Table=aDr.CYDr  InternalRulePriority=Speed  RndMeth=Simplest
  2-D Lookup Table4 : Lookup_n-D  NumberOfTableDimensions=1  BreakpointsForDimension1=aDr.alpha  BreakpointsForDimension2=aDe.alpha  BreakpointsForDimension3=aDe.flap  Table=aDr.ClDr  InternalRulePriority=Speed  RndMeth=Simplest
  2-D Lookup Table5 : Lookup_n-D  NumberOfTableDimensions=1  BreakpointsForDimension1=aDr.alpha  BreakpointsForDimension2=aDe.alpha  BreakpointsForDimension3=aDe.flap  Table=aDr.CnDr  InternalRulePriority=Speed  RndMeth=Simplest
  Divide{,1..5} (6 alike) : Product  Inputs=**
  Mux1 : Mux  Inputs=6
  dr_Coeff : Outport  VectorParamsAs1DForOutWhenUnconnected=off
  wires:
  dr/1 -> Divide5/1, Divide4/1, Divide3/1, Divide2/1, Divide1/1, Divide/1
  alpha/1 -> 2-D Lookup Table5/1, 2-D Lookup Table1/1, 2-D Lookup Table4/1, 2-D Lookup Table3/1, 2-D Lookup Table2/1, 2-D Lookup Table/1
  Divide/1 -> Mux1/1
  2-D Lookup Table5/1 -> Divide5/2
  Divide5/1 -> Mux1/6
  2-D Lookup Table1/1 -> Divide4/2
  Divide4/1 -> Mux1/5
  Divide2/1 -> Mux1/3
  2-D Lookup Table4/1 -> Divide3/2
  2-D Lookup Table/1 -> Divide/2
  2-D Lookup Table3/1 -> Divide2/2
  Mux1/1 -> dr_Coeff/1
  Divide3/1 -> Mux1/4
  2-D Lookup Table2/1 -> Divide1/2
  Divide1/1 -> Mux1/2

== system eVTOL_HIL/eVTOL Dynamic Model/Environment/Wind Models/Dryden Wind Turbulence Model (Continuous (+q -r))/Select angular rates/Interpolate rates/wind to body transformation/convert to earth coords ==
  Wind direction : Inport
  pg_l : Inport  Port=2
  qg_l : Inport  Port=3
  Demux : Demux  Outputs=2
      settings: DisplayOption=none
  Demux1 : Demux  Outputs=2
      settings: DisplayOption=none
  Mux : Mux  Inputs=2
  Mux1 : Mux  Inputs=2
  Product1 : Product  InputSameDT=on  SaturateOnIntegerOverflow=on  OutDataTypeStr=Inherit: Same as first input
  Product2 : Product  InputSameDT=on  SaturateOnIntegerOverflow=on  OutDataTypeStr=Inherit: Same as first input
  Selector : Selector  InputPortWidth=4  IndexOptions=Index vector (dialog)  Indices=[1 4]  OutputSizes=1
  Selector1 : Selector  InputPortWidth=4  IndexOptions=Index vector (dialog)  Indices=[2 3]  OutputSizes=1
  Sum : Sum  Inputs=|+-  SaturateOnIntegerOverflow=on
  Sum1 : Sum  Inputs=|++  SaturateOnIntegerOverflow=on
  Trigonometric Function : Trigonometry  Operator=sincos
  pg : Outport  VectorParamsAs1DForOutWhenUnconnected=off
  qg : Outport  Port=2  VectorParamsAs1DForOutWhenUnconnected=off
  wires:
  Trigonometric Function/1 -> Product1/1
  Trigonometric Function/2 -> Product2/2
  Selector1/1 -> Demux1/1
  Selector/1 -> Demux/1
  Mux1/1 -> Selector1/1, Selector/1
  Product1/1 -> Mux1/2
  Product2/1 -> Mux1/1
  Demux1/2 -> Sum1/2
  Demux1/1 -> Sum1/1
  Demux/2 -> Sum/2
  Demux/1 -> Sum/1
  Sum1/1 -> qg/1
  Sum/1 -> pg/1
  Mux/1 -> Product2/1, Product1/2
  qg_l/1 -> Mux/2
  pg_l/1 -> Mux/1
  Wind direction/1 -> Trigonometric Function/1

== system eVTOL_HIL/eVTOL Dynamic Model/Environment/Wind Models/Dryden Wind Turbulence Model (Continuous (+q -r))/Select angular rates/Low altitude rates/wind to body transformation/convert to earth coords ==
  Wind direction : Inport
  pg_l : Inport  Port=2
  qg_l : Inport  Port=3
  Demux : Demux  Outputs=2
      settings: DisplayOption=none
  Demux1 : Demux  Outputs=2
      settings: DisplayOption=none
  Mux : Mux  Inputs=2
  Mux1 : Mux  Inputs=2
  Product1 : Product  InputSameDT=on  SaturateOnIntegerOverflow=on  OutDataTypeStr=Inherit: Same as first input
  Product2 : Product  InputSameDT=on  SaturateOnIntegerOverflow=on  OutDataTypeStr=Inherit: Same as first input
  Selector : Selector  InputPortWidth=4  IndexOptions=Index vector (dialog)  Indices=[1 4]  OutputSizes=1
  Selector1 : Selector  InputPortWidth=4  IndexOptions=Index vector (dialog)  Indices=[2 3]  OutputSizes=1
  Sum : Sum  Inputs=|+-  SaturateOnIntegerOverflow=on
  Sum1 : Sum  Inputs=|++  SaturateOnIntegerOverflow=on
  Trigonometric Function1 : Trigonometry  Operator=sincos
  pg : Outport  VectorParamsAs1DForOutWhenUnconnected=off
  qg : Outport  Port=2  VectorParamsAs1DForOutWhenUnconnected=off
  wires:
  Trigonometric Function1/2 -> Product2/2
  Wind direction/1 -> Trigonometric Function1/1
  pg_l/1 -> Mux/1
  qg_l/1 -> Mux/2
  Trigonometric Function1/1 -> Product1/1
  Mux/1 -> Product1/2, Product2/1
  Sum/1 -> pg/1
  Sum1/1 -> qg/1
  Demux/1 -> Sum/1
  Demux/2 -> Sum/2
  Demux1/1 -> Sum1/1
  Demux1/2 -> Sum1/2
  Product2/1 -> Mux1/1
  Product1/1 -> Mux1/2
  Mux1/1 -> Selector/1, Selector1/1
  Selector/1 -> Demux/1
  Selector1/1 -> Demux1/1

== system eVTOL_HIL/eVTOL Dynamic Model/Environment/Wind Models/Dryden Wind Turbulence Model (Continuous (+q -r))/Select velocities/Interpolate velocities/wind to body transformation/convert to earth coords ==
  Wind direction : Inport
  ug_l : Inport  Port=2
  vg_l : Inport  Port=3
  Demux : Demux  Outputs=2
      settings: DisplayOption=none
  Demux1 : Demux  Outputs=2
      settings: DisplayOption=none
  Mux : Mux  Inputs=2
  Mux1 : Mux  Inputs=2
  Product1 : Product  InputSameDT=on  SaturateOnIntegerOverflow=on  OutDataTypeStr=Inherit: Same as first input
  Product2 : Product  InputSameDT=on  SaturateOnIntegerOverflow=on  OutDataTypeStr=Inherit: Same as first input
  Selector : Selector  InputPortWidth=4  IndexOptions=Index vector (dialog)  Indices=[1 4]  OutputSizes=1
  Selector1 : Selector  InputPortWidth=4  IndexOptions=Index vector (dialog)  Indices=[2 3]  OutputSizes=1
  Sum : Sum  Inputs=|+-  SaturateOnIntegerOverflow=on
  Sum1 : Sum  Inputs=|++  SaturateOnIntegerOverflow=on
  Trigonometric Function : Trigonometry  Operator=sincos
  ug : Outport  VectorParamsAs1DForOutWhenUnconnected=off
  vg : Outport  Port=2  VectorParamsAs1DForOutWhenUnconnected=off
  wires:
  Trigonometric Function/2 -> Product2/2
  Wind direction/1 -> Trigonometric Function/1
  ug_l/1 -> Mux/1
  vg_l/1 -> Mux/2
  Trigonometric Function/1 -> Product1/1
  Mux/1 -> Product1/2, Product2/1
  Sum/1 -> ug/1
  Sum1/1 -> vg/1
  Demux/1 -> Sum/1
  Demux/2 -> Sum/2
  Demux1/1 -> Sum1/1
  Demux1/2 -> Sum1/2
  Product2/1 -> Mux1/1
  Product1/1 -> Mux1/2
  Mux1/1 -> Selector/1, Selector1/1
  Selector/1 -> Demux/1
  Selector1/1 -> Demux1/1

== system eVTOL_HIL/eVTOL Dynamic Model/Environment/Wind Models/Dryden Wind Turbulence Model (Continuous (+q -r))/Select velocities/Low altitude velocities/wind to body transformation/convert to earth coords ==
  Wind direction : Inport
  ug_l : Inport  Port=2
  vg_l : Inport  Port=3
  Demux : Demux  Outputs=2
      settings: DisplayOption=none
  Demux1 : Demux  Outputs=2
      settings: DisplayOption=none
  Mux : Mux  Inputs=2
  Mux1 : Mux  Inputs=2
  Product1 : Product  InputSameDT=on  SaturateOnIntegerOverflow=on  OutDataTypeStr=Inherit: Same as first input
  Product2 : Product  InputSameDT=on  SaturateOnIntegerOverflow=on  OutDataTypeStr=Inherit: Same as first input
  Selector : Selector  InputPortWidth=4  IndexOptions=Index vector (dialog)  Indices=[1 4]  OutputSizes=1
  Selector1 : Selector  InputPortWidth=4  IndexOptions=Index vector (dialog)  Indices=[2 3]  OutputSizes=1
  Sum : Sum  Inputs=|+-  SaturateOnIntegerOverflow=on
  Sum1 : Sum  Inputs=|++  SaturateOnIntegerOverflow=on
  Trigonometric Function : Trigonometry  Operator=sincos
  ug : Outport  VectorParamsAs1DForOutWhenUnconnected=off
  vg : Outport  Port=2  VectorParamsAs1DForOutWhenUnconnected=off
  wires:
  Trigonometric Function/2 -> Product2/2
  Selector1/1 -> Demux1/1
  Selector/1 -> Demux/1
  Mux1/1 -> Selector1/1, Selector/1
  Product1/1 -> Mux1/2
  Product2/1 -> Mux1/1
  Demux1/2 -> Sum1/2
  Demux1/1 -> Sum1/1
  Demux/2 -> Sum/2
  Demux/1 -> Sum/1
  Sum1/1 -> vg/1
  Sum/1 -> ug/1
  Mux/1 -> Product2/1, Product1/2
  Trigonometric Function/1 -> Product1/1
  vg_l/1 -> Mux/2
  ug_l/1 -> Mux/1
  Wind direction/1 -> Trigonometric Function/1

== matlab function eVTOL_HIL/eVTOL Dynamic Model/hil_state_quaternion_pack1/payload_hil_state_quaternion/MATLAB Function ==
  data: dcm input; q output
function q = fcn(dcm)
% DCM 应该是一个 3x3 的方向余弦矩阵 (旋转矩阵)
% q 输出是一个 4x1 的四元数 [q0; q1; q2; q3] (即 [w; x; y; z])

    q = zeros(4,1);
    tr = trace(dcm);
    
    if tr > 0
        S = sqrt(tr + 1.0) * 2; 
        q(1) = 0.25 * S;
        q(2) = (dcm(3,2) - dcm(2,3)) / S;
        q(3) = (dcm(1,3) - dcm(3,1)) / S;
        q(4) = (dcm(2,1) - dcm(1,2)) / S;
    elseif (dcm(1,1) > dcm(2,2)) && (dcm(1,1) > dcm(3,3))
        S = sqrt(1.0 + dcm(1,1) - dcm(2,2) - dcm(3,3)) * 2;
        q(1) = (dcm(3,2) - dcm(2,3)) / S;
        q(2) = 0.25 * S;
        q(3) = (dcm(1,2) + dcm(2,1)) / S;
        q(4) = (dcm(1,3) + dcm(3,1)) / S;
    elseif dcm(2,2) > dcm(3,3)
        S = sqrt(1.0 + dcm(2,2) - dcm(1,1) - dcm(3,3)) * 2;
        q(1) = (dcm(1,3) - dcm(3,1)) / S;
        q(2) = (dcm(1,2) + dcm(2,1)) / S;
        q(3) = 0.25 * S;
        q(4) = (dcm(2,3) + dcm(3,2)) / S;
    else
        S = sqrt(1.0 + dcm(3,3) - dcm(1,1) - dcm(2,2)) * 2;
        q(1) = (dcm(2,1) - dcm(1,2)) / S;
        q(2) = (dcm(1,3) + dcm(3,1)) / S;
        q(3) = (dcm(2,3) + dcm(3,2)) / S;
        q(4) = 0.25 * S;
    end
end

== matlab function eVTOL_HIL/eVTOL Dynamic Model/airframe/Flight Conditions/MATLAB Function ==
  data: u input; y output
function y = fcn(u)
    y = norm(u);
end
